simulink model "Requriment1"  (R2021a)
settings: Solver=FixedStepDiscrete  StartTime=0.0  StopTime=50  FixedStep=1  RelTol=1e-3
libraries: simulink x2
settings Model: Creator=Admin  LastModifiedBy=Rahul
settings SolverCC: AlgebraicLoopSolver=TrustRegion
settings DataIOCC: InspectSignalLogs=on  SignalLoggingName=mil_out  LoggingToFile=on  LoggingFileName=mil_out.mat
settings OptimizationCC: DefaultParameterBehavior=Inlined  UseDivisionForNetSlopeComputation=on  GainParamInheritBuiltInType=on  UseFloatMulNetSlope=on  InlineInvariantSignals=on  PassReuseOutputArgsAs=Individual arguments  ZeroExternalMemoryAtStartup=off  ZeroInternalMemoryAtStartup=off  NoFixptDivByZeroProtection=on  EfficientFloat2IntCast=on  LifeSpan=1  OptimizeBlockOrder=speed  DifferentSizesBufferReuse=on  EfficientTunableParamExpr=on
settings DebuggingCC: SignalInfNanChecking=error  ParameterTunabilityLossMsg=error  UniqueDataStoreMsg=error  AssertControl=DisableAll  StrictBusMsg=ErrorOnBusTreatedAsVector  SFUndirectedBroadcastEventsDiag=error  SFMachineParentedDataDiag=warning
settings HardwareCC: ProdLongLongMode=on
settings SFSimCC: CompileTimeRecursionLimit=0  EnableRuntimeRecursion=off  MATLABDynamicMemAlloc=off  CustomCodeUndefinedFunction=UseInterfaceOnly
settings RTWCC: SystemTargetFile=ert.tlc  TemplateMakefile=ert_default_tmf  GenerateReport=on  IncludeHyperlinkInReport=on  LaunchReport=on  GenerateTraceInfo=on  GenerateTraceReport=on  GenerateTraceReportSl=on  GenerateTraceReportSf=on  GenerateTraceReportEml=on  GenerateCodeMetricsReport=on
settings CodeAppCC: ForceParamTrailComments=on  IgnoreCustomStorageClasses=off  OperatorAnnotations=on  SimulinkDataObjDesc=on  SFDataObjDesc=on  MATLABFcnDesc=on  CustomSymbolStrGlobalVar=rt$N$M  CustomSymbolStrType=$N$M  CustomSymbolStrFcn=$N$M$F  CustomSymbolStrMacro=$N$M  InsertBlockDesc=on
settings ERTTargetCC: TargetLangStandard=C99 (ISO)  UtilityFuncGeneration=Shared location  GenerateSampleERTMain=on  IncludeMdlTerminateFcn=off  CombineSignalStateStructs=on  SuppressErrorStatus=on  SupportAbsoluteTime=off  SupportNonFinite=off  SupportComplex=off  ParenthesesLevel=Maximum  CastingMode=Standards  GenerateSharedConstants=off  InlinedParameterPlacement=NonHierarchical  ERTCustomFileTemplate=example_file_process.tlc  ERTFilePackagingFormat=CompactWithDataFile  EnableSignedLeftShifts=off  EnableSignedRightShifts=off
settings ConfigComp: CovMetricSettings=dcmwe

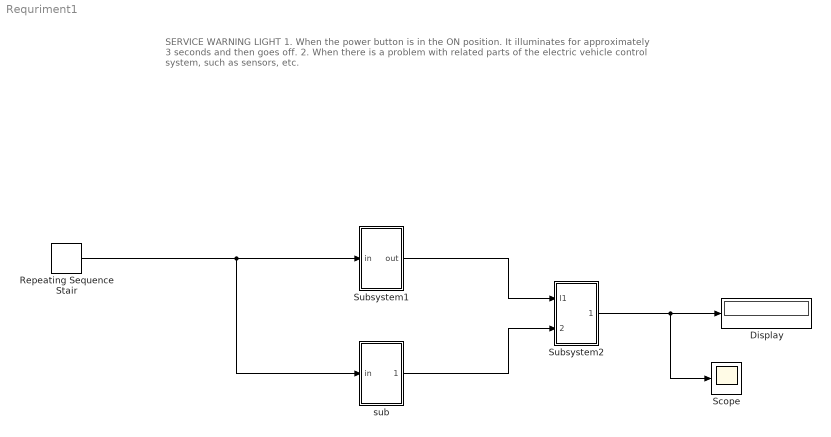
== system Requriment1 ==
  note: SERVICE WARNING LIGHT
      | 1. When the power button is in the ON position.
      | It illuminates for approximately 3 seconds and then goes off.
      | 2. When there is a problem with related parts of the electric vehicle control system, such as sensors, etc.
  Display : Display
  Repeating Sequence Stair : simulink/Sources/Repeating Sequence Stair  OutValues=[1 1 1 1 0 0 0 1 1 1 1 0 0 0]  tsamp=-1  OutMin=[]  OutMax=[]  OutDataTypeStr=double  OutputDataTypeScalingMode=double  OutDataType=fixdt(0,8)  ConRadixGroup=Best Precision: Vector-wise  OutScaling=2^-12
  Scope : Scope
  Subsystem1 : Subsystem
  Subsystem2 : Subsystem
  sub : Subsystem
  wires:
  Repeating Sequence Stair/1 -> sub/1(in), Subsystem1/1(in)
  Subsystem2/1(out) -> Scope/1, Display/1
  sub/1(Out1) -> Subsystem2/2(In2)
  Subsystem1/1(out) -> Subsystem2/1(l1)

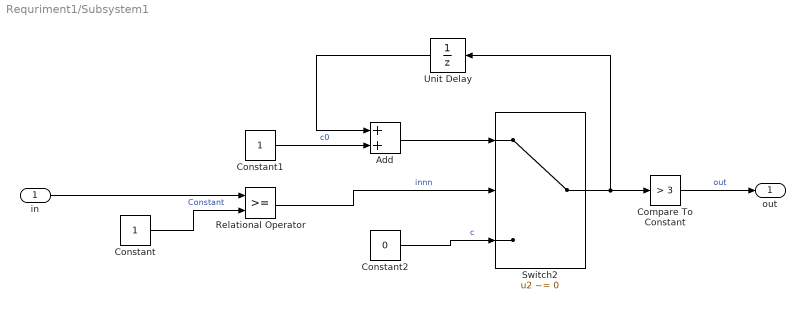
== system Requriment1/Subsystem1 ==
  in : Inport
  Add : Sum
  Compare To Constant : simulink/Logic and Bit Operations/Compare To Constant  relop=>  const=3  OutDataTypeStr=boolean
  Constant : Constant
  Constant1 : Constant
  Constant2 : Constant  Value=0
  Relational Operator : RelationalOperator  OutDataTypeStr=boolean  RndMeth=Simplest
  Switch2 : Switch  Criteria=u2 ~= 0
  Unit Delay : UnitDelay  SampleTime=-1  HasFrameUpgradeWarning=on
  out : Outport  VectorParamsAs1DForOutWhenUnconnected=off
  wires:
  in/1 -> Relational Operator/1
  Constant/1 -> Relational Operator/2  "Constant"
  Unit Delay/1 -> Add/1
  Constant2/1 -> Switch2/3  "c"
  Switch2/1 -> Unit Delay/1, Compare To Constant/1
  Constant1/1 -> Add/2  "c0"
  Add/1 -> Switch2/1
  Compare To Constant/1 -> out/1  "out"
  Relational Operator/1 -> Switch2/2  "innn"

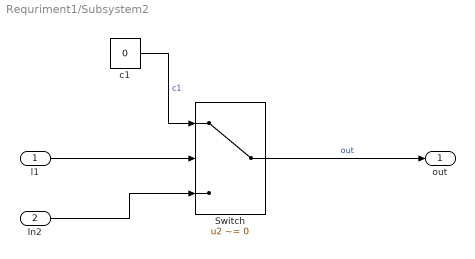
== system Requriment1/Subsystem2 ==
  l1 : Inport
  In2 : Inport  Port=2
  Switch : Switch  Criteria=u2 ~= 0
  c1 : Constant  Value=0
  out : Outport  VectorParamsAs1DForOutWhenUnconnected=off
  wires:
  l1/1 -> Switch/2
  c1/1 -> Switch/1  "c1"
  Switch/1 -> out/1  "out"
  In2/1 -> Switch/3

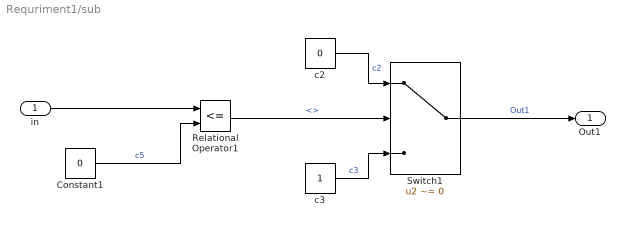
== system Requriment1/sub ==
  in : Inport
  Constant1 : Constant  Value=0
  Relational Operator1 : RelationalOperator  Operator=<=  OutDataTypeStr=boolean  RndMeth=Simplest
  Switch1 : Switch  Criteria=u2 ~= 0
  c2 : Constant  Value=0
  c3 : Constant
  Out1 : Outport  VectorParamsAs1DForOutWhenUnconnected=off
  wires:
  c3/1 -> Switch1/3  "c3"
  c2/1 -> Switch1/1  "c2"
  in/1 -> Relational Operator1/1
  Relational Operator1/1 -> Switch1/2  "<>"
  Constant1/1 -> Relational Operator1/2  "c5"
  Switch1/1 -> Out1/1  "Out1"
